simulink model "cl_ctorque"  (R2024b)
settings: Solver=VariableStepAuto  StartTime=0.0  StopTime=Tmax  RelTol=1e-3
values from neighbouring files (symbols this model uses):
  Kd = 2    [controlled_robot_def_ctorque.m]    (also in controlled_robot_def_freedfwrd.m = [5])
  Kp = [50 50 50]    [controlled_robot_def_Nested.m]    (also in controlled_robot_def_ctorque.m = 20; controlled_robot_def_freedfwrd.m = [100])
  q_inicial = [0 0 0]    [circle_drawing.m]    (also in controlled_robot_def_Nested.m; controlled_robot_def_PD.m; controlled_robot_def_PID.m; controlled_robot_def_ctorque.m)
  robot_3dof = SerialLink(L, 'name', 'Robot 3-DOF')    [circle_drawing.m]    (also in controlled_robot_def_Nested.m; controlled_robot_def_PD.m; controlled_robot_def_PID.m; controlled_robot_def_ctorque.m)
  Tm = Ts_calculated    [controlled_robot_def_Nested.m]    (also in controlled_robot_def_PD.m; controlled_robot_def_PID.m; controlled_robot_def_ctorque.m; controlled_robot_def_freedfwrd.m)
  unc = 0.2    [controlled_robot_def_Nested.m]    (also in controlled_robot_def_PD.m; controlled_robot_def_PID.m = 0; controlled_robot_def_ctorque.m; controlled_robot_def_freedfwrd.m)
undefined symbols (not defined in the file or in its folder): slcoulomb
libraries: roblocks x2
settings Model: Creator=pablo  LastModifiedBy=pablo

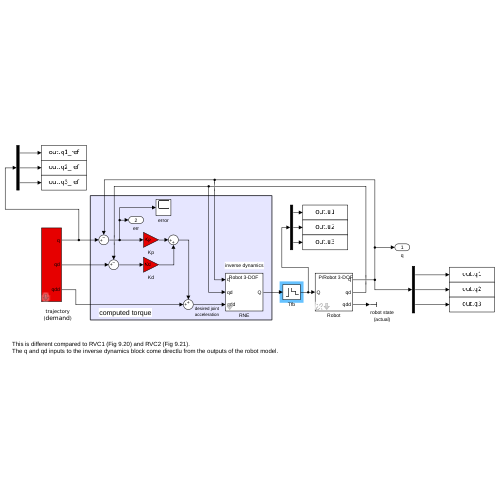
[thumbnail: Simulink's stored preview of the top-level diagram]
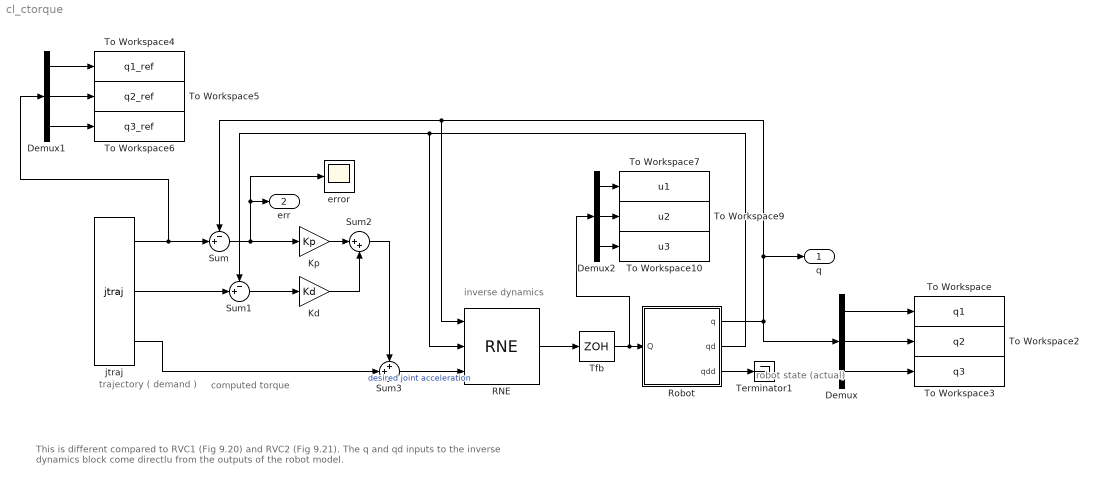
== system cl_ctorque ==
  note: trajectory
      | ( demand )
  note: This is different compared to RVC1 (Fig 9.20) and RVC2 (Fig 9.21).
      | The q and qd inputs to the inverse dynamics block come directlu from the outputs of the robot model.
  note: inverse dynamics
  note: computed torque
  note: robot state
      | (actual)
  Demux : Demux  Outputs=3
  Demux1 : Demux  Outputs=3
  Demux2 : Demux  Outputs=3
  Kd : Gain  Gain=Kd  SaturateOnIntegerOverflow=on  OutDataTypeStr=Inherit: Same as input  ParamDataTypeStr=Inherit: Same as input
  Kp : Gain  Gain=Kp  SaturateOnIntegerOverflow=on  OutDataTypeStr=Inherit: Same as input  ParamDataTypeStr=Inherit: Same as input
  RNE : roblocks/Arm/RNE  robot=robot_3dof  grav=[0 0 9.81]
  Robot : Subsystem  AncestorBlock=roblocks/Arm/Robot  mask{robot=robot_3dof.perturb(unc), q0=q_inicial}
      mask prompts: robot "Robot object"; q0 "Initial state"
      mask help: Rigid-body dynamic model of robot.
      mask init:
      | if isa(robot, 'SerialLink')
      |     rname = robot.name;
      |     %fprintf('**robot name is %s\n', rname);
      | else
      |     rname = '';
      |     n = 0
      | end
      mask Help:
      | Simulates the forward (direct) rigid-body dynamics of the robot described
      | by the given robot object.  For given applied joint torque/force it computes
      | the instaneous joint coordinates, velocities and acclerations.
      | 
      | 
      | <b>Parameters::</b>
      | 
      | robot (SerialLink) a dynamic model of an N-link serial link manipulator
      | q0 (1xN)  Initial joint coordinates
      | 
      | <b>Inputs::</b>
      | 
      | Q (1xN) the generalized joint force (torque or force) required to achieve
      | the motion state (q, qd, qdd).
      | 
      | <b>Outputs::</b>
      | 
      | q (1xN) joint coordinates
      | qd (1xN) joint coordinate velocity
      | qdd (1xN) joint coordinate acceleration
      | 
      | 
      | <b>Notes::</b>
      | 
      | - Required to simulate robot rigid body motion.
      | - Implemented using the recursive Newton-Euler scheme (RNE).
      | - A wrapper for the Toolbox method accel() which in turn depends on the
      |   method rne().
      mask Display:
      | port_label('input', 1, 'Q')
      | port_label('output', 1, 'q')
      | port_label('output', 2, 'qd')
      | port_label('output', 3, 'qdd')
      | text(0.1, 0.9,  rname, 'horizontalAlignment', 'left')
  Sum : Sum  Inputs=-+|  InputSameDT=on  SaturateOnIntegerOverflow=on  OutDataTypeStr=Inherit: Same as first input
  Sum1 : Sum  Inputs=-+|  InputSameDT=on  SaturateOnIntegerOverflow=on  OutDataTypeStr=Inherit: Same as first input
  Sum2 : Sum  Inputs=|++  InputSameDT=on  SaturateOnIntegerOverflow=on  OutDataTypeStr=Inherit: Same as first input
  Sum3 : Sum  Inputs=++|  InputSameDT=on  SaturateOnIntegerOverflow=on  OutDataTypeStr=Inherit: Same as first input
  Terminator1 : Terminator
  Tfb : ZeroOrderHold  SampleTime=Tm
  To Workspace : ToWorkspace  VariableName=q1  SaveFormat=Timeseries  SampleTime=-1
  To Workspace10 : ToWorkspace  VariableName=u3  SaveFormat=Timeseries  SampleTime=-1
  To Workspace2 : ToWorkspace  VariableName=q2  SaveFormat=Timeseries  SampleTime=-1
  To Workspace3 : ToWorkspace  VariableName=q3  SaveFormat=Timeseries  SampleTime=-1
  To Workspace4 : ToWorkspace  VariableName=q1_ref  SaveFormat=Timeseries  SampleTime=-1
  To Workspace5 : ToWorkspace  VariableName=q2_ref  SaveFormat=Timeseries  SampleTime=-1
  To Workspace6 : ToWorkspace  VariableName=q3_ref  SaveFormat=Timeseries  SampleTime=-1
  To Workspace7 : ToWorkspace  VariableName=u1  SaveFormat=Timeseries  SampleTime=-1
  To Workspace9 : ToWorkspace  VariableName=u2  SaveFormat=Timeseries  SampleTime=-1
  error : Scope
  jtraj : roblocks/Toolbox/jtraj  q0=q_inicial  qf=qf  tmax=Tmax  ts=-1
  q : Outport  VectorParamsAs1DForOutWhenUnconnected=off
  err : Outport  Port=2  VectorParamsAs1DForOutWhenUnconnected=off
  wires:
  jtraj/3 -> Sum3/2
  Tfb/1 -> Demux2/1, Robot/1(Q)
  Sum3/1 -> RNE/3  "desired joint acceleration"
  Robot/2(qd) -> RNE/2, Sum1/1
  jtraj/2 -> Sum1/2
  jtraj/1 -> Demux1/1, Sum/2
  RNE/1 -> Tfb/1
  Robot/3(qdd) -> Terminator1/1
  Kd/1 -> Sum2/2
  Sum1/1 -> Kd/1
  Sum/1 -> error/1, err/1, Kp/1
  Robot/1(q) -> q/1, RNE/1, Sum/1, Demux/1
  Sum2/1 -> Sum3/1
  Kp/1 -> Sum2/1
  Demux/1 -> To Workspace/1
  Demux/2 -> To Workspace2/1
  Demux/3 -> To Workspace3/1
  Demux1/1 -> To Workspace4/1
  Demux1/2 -> To Workspace5/1
  Demux1/3 -> To Workspace6/1
  Demux2/1 -> To Workspace7/1
  Demux2/2 -> To Workspace9/1
  Demux2/3 -> To Workspace10/1

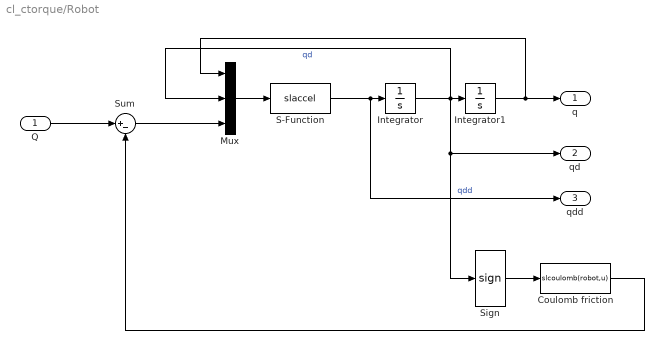
== system cl_ctorque/Robot ==
  Q : Inport
  Coulomb friction : MATLABFcn  MATLABFcn=slcoulomb(robot,u)  OutputDimensions=[robot.n 1]  Output1D=off
  Integrator : Integrator
  Integrator1 : Integrator  InitialCondition=q0
  Mux : Mux  Inputs=3
  S-Function : S-Function  FunctionName=slaccel  Parameters=robot  SFunctionDeploymentMode=off  EnableBusSupport=off
  Sign : Signum
  Sum : Sum  Inputs=|+-
  q : Outport  VectorParamsAs1DForOutWhenUnconnected=off
  qd : Outport  Port=2  VectorParamsAs1DForOutWhenUnconnected=off
  qdd : Outport  Port=3  VectorParamsAs1DForOutWhenUnconnected=off
  wires:
  S-Function/1 -> qdd/1, Integrator/1  "qdd"
  Mux/1 -> S-Function/1
  Integrator/1 -> Sign/1, qd/1, Integrator1/1, Mux/2  "qd"
  Integrator1/1 -> q/1, Mux/1
  Q/1 -> Sum/1
  Sum/1 -> Mux/3
  Coulomb friction/1 -> Sum/2
  Sign/1 -> Coulomb friction/1
